simulink model "LPV_controller_Simulation_6DOF"  (R2015a)
settings: Solver=ode1  StartTime=0.0  StopTime=1.5  FixedStep=0.001  RelTol=1e-3
undefined symbols (not defined in the file): dKLFR_sim, inert, phi_mid, phi_range, rho_bnd, robot3DOFaffineLPVparams, theta_bnd, theta_mid, theta_range, Xdsim
libraries: simulink x4
settings Model: Creator=Micha  LastModifiedBy=Micha

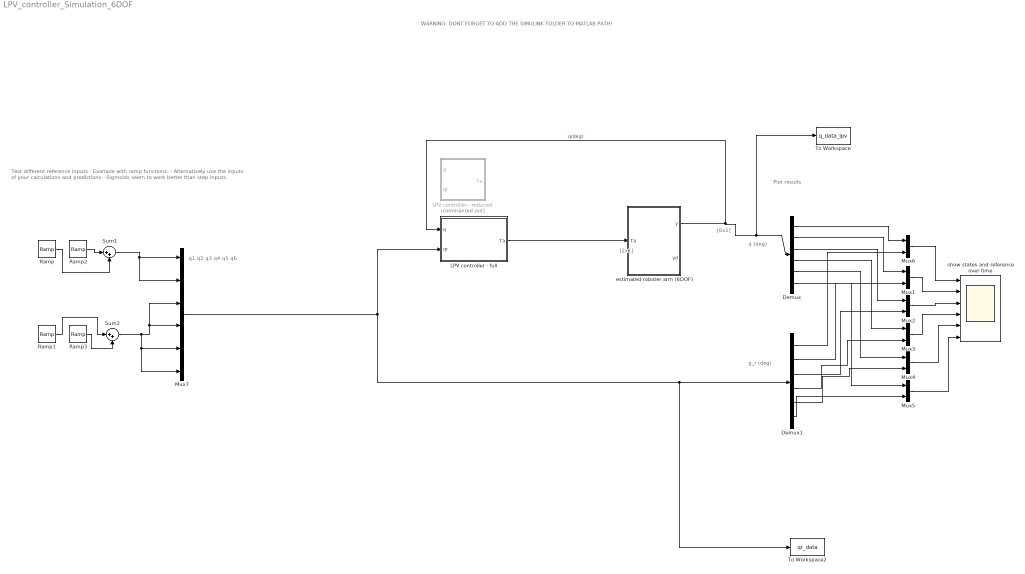
== system LPV_controller_Simulation_6DOF ==
  note: WARNING: DONT FORGET TO ADD THE SIMULINK FOLDER TO MATLAB PATH!
  note: Test different reference inputs - Example with ramp functions.
      | - Alternatively use the inputs of your calculations and predictions
      | - Sigmoids seem to work better than step inputs.
  note: [6x1]
  note: Plot results
  note: g_r (deg)
  note: [2x1]
  note: q (deg)
  note: q1
      |
      |
      | q2
      |
      |
      |
      | q3
      |
      |
      |
      |
      | q4
      |
      |
      |
      | q5
      |
      |
      |
      | q6
  Demux : Demux  Outputs=6
  Demux1 : Demux  Outputs=6
  LPV controller - full : Subsystem
  LPV controller - reduced : Subsystem  Commented=on
  Mux{1..6} (6 alike) : Mux  Inputs=2
  Mux7 : Mux  Inputs=6
  Ramp : simulink/Sources/Ramp  slope=-80  start=0.1  X0=0
  Ramp1 : simulink/Sources/Ramp  slope=60  start=0.1  X0=0
  Ramp2 : simulink/Sources/Ramp  slope=80  start=0.6  X0=0
  Ramp3 : simulink/Sources/Ramp  slope=-60  start=1  X0=0
  Sum1 : Sum  Inputs=|++
  Sum2 : Sum  Inputs=|++
  To Workspace : ToWorkspace  VariableName=q_data_lpv  SaveFormat=Timeseries  SampleTime=-1
  To Workspace2 : ToWorkspace  VariableName=qr_data  SaveFormat=Timeseries  SampleTime=-1
  "estimated roboter arm (6DOF) " : Subsystem
  show states and reference over time : Scope  NumInputPorts=6
      settings: YMin=-45~-45~10~5~5~5  YMax=-10~-10~55~55~55~55
  wires:
  Demux/1 -> Mux6/1
  Demux/2 -> Mux1/1
  Demux/3 -> Mux2/1
  Demux/4 -> Mux3/1
  Demux/5 -> Mux4/1
  Demux/6 -> Mux5/1
  Mux6/1 -> show states and reference over time/1
  Mux1/1 -> show states and reference over time/2
  Mux2/1 -> show states and reference over time/3
  Mux3/1 -> show states and reference over time/4
  Mux4/1 -> show states and reference over time/5
  Mux5/1 -> show states and reference over time/6
  Demux1/1 -> Mux6/2
  Demux1/2 -> Mux1/2
  Demux1/3 -> Mux2/2
  Demux1/4 -> Mux3/2
  Demux1/5 -> Mux4/2
  Demux1/6 -> Mux5/2
  Mux7/1 -> Demux1/1, To Workspace2/1, LPV controller - full/2(qr)
  LPV controller - full/1(Ta) -> "estimated roboter arm (6DOF) "/1(Ta)
  Ramp2/1 -> Sum1/1
  Ramp/1 -> Sum1/2
  Ramp1/1 -> Sum2/1
  Ramp3/1 -> Sum2/2
  Sum2/1 -> Mux7/6, Mux7/5, Mux7/4, Mux7/3
  Sum1/1 -> Mux7/1, Mux7/2
  "estimated roboter arm (6DOF) "/1(y) -> To Workspace/1, Demux/1, LPV controller - full/1(q)  "q(deg)"

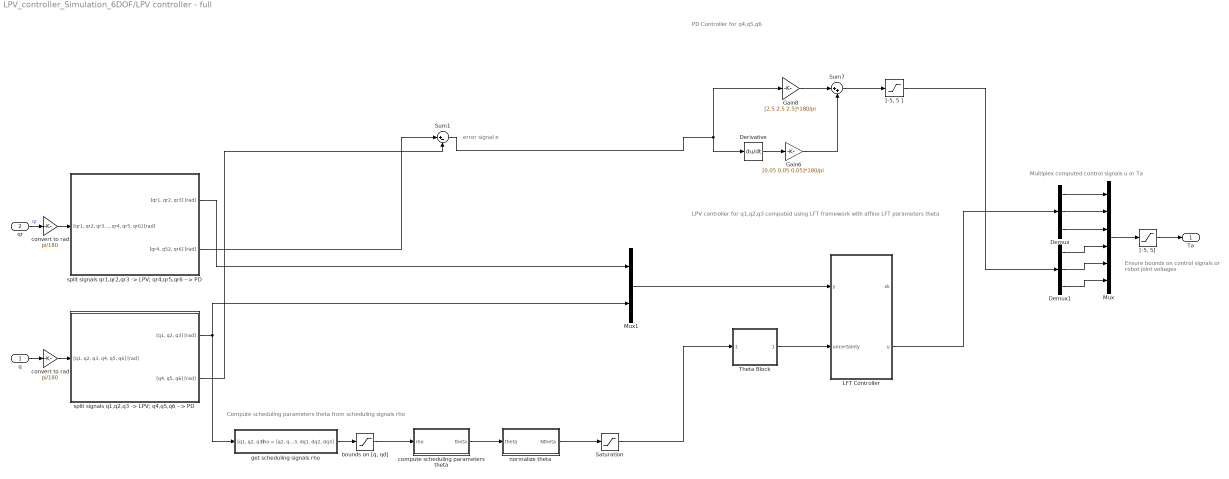
== system LPV_controller_Simulation_6DOF/LPV controller - full ==
  note: Ensure bounds on control signals
      |  or robot joint voltages
  note: Multiplex computed control signals u or Ta
  note: Compute scheduling parameters theta from scheduling signals rho
  note: error signal e
  note: LPV controller for q1,q2,q3 computed using LFT framework
      | with affine LFT parameters theta
  note: PD Controller for q4,q5,q6
  q : Inport
  qr : Inport  Port=2
  Demux : Demux  Outputs=3
  Demux1 : Demux  Outputs=3
  Derivative : Derivative
  Gain6 : Gain  Gain=[0.05 0.05 0.05]*180/pi
      settings: AttributesFormatString=D gain
  Gain8 : Gain  Gain=[2.5 2.5 2.5]*180/pi
      settings: AttributesFormatString=P gain
  LFT Controller : Subsystem  mask{P=dKLFR_sim}
      mask prompts: P "Plant"
      mask Display:
      | port_label('output', 1, 'xk')
      | port_label('output', 2, 'u')
      | port_label('input' , 1, 'e')
      | port_label('input' , 2, 'phi')
      | fprintf('Controller')
  Mux : Mux  Inputs=6
  Mux1 : Mux  Inputs=2
  Saturation : Saturate  UpperLimit=1  LowerLimit=-1
  Sum1 : Sum  Inputs=|+-
  Sum7 : Sum  Inputs=|++
  Theta Block : Subsystem
      mask Display:
      | patch([0.2 .5 0.8], [0.2 0.8 0.2], [0 0 0])
      | patch([0.25 .5 0.75], [0.25 0.75 0.25], [1 1 1])
  "[-5, 5 ]" : Saturate  UpperLimit=5  LowerLimit=-5
  "[-5, 5]" : Saturate  UpperLimit=5  LowerLimit=-5
  "bounds on [q, qd]" : Saturate  UpperLimit=rho_bnd(:, 2)  LowerLimit=rho_bnd(:, 1)
  compute scheduling parameters theta : Subsystem
  convert to rad : Gain  Gain=pi/180
  convert to rad : Gain  Gain=pi/180
  get scheduling signals rho : Subsystem
  normalize theta : Subsystem
  "split signals q1,q2,q3 -> LPV; q4,q5,q6 --> PD" : Subsystem
  "split signals qr1,qr2,qr3 -> LPV; qr4,qr5,qr6 --> PD" : Subsystem
  Ta : Outport
  wires:
  q/1 -> convert to rad/1
  qr/1 -> convert to rad/1  "qr"
  convert to rad/1 -> "split signals q1,q2,q3 -> LPV; q4,q5,q6 --> PD"/1("[q1, q2, q3, q4, q5, q6] [rad]")
  convert to rad/1 -> "split signals qr1,qr2,qr3 -> LPV; qr4,qr5,qr6 --> PD"/1("[qr1, qr2, qr3, qr4, qr5, qr6] [rad]")
  "split signals q1,q2,q3 -> LPV; q4,q5,q6 --> PD"/1("[q1, q2, q3] [rad]") -> get scheduling signals rho/1("[q1, q2, q3]"), Mux1/2
  LFT Controller/2(u) -> Demux/1
  Mux1/1 -> LFT Controller/1(y)
  Demux/1 -> Mux/1
  Demux/2 -> Mux/2
  "split signals qr1,qr2,qr3 -> LPV; qr4,qr5,qr6 --> PD"/1("[qr1, qr2, qr3] [rad]") -> Mux1/1
  get scheduling signals rho/1("rho = [q2, q3, dq1, dq2, dq3]") -> "bounds on [q, qd]"/1
  Saturation/1 -> Theta Block/1(Scheduling Parameter Vector)
  "bounds on [q, qd]"/1 -> compute scheduling parameters theta/1(rho)
  Mux/1 -> "[-5, 5]"/1
  "[-5, 5]"/1 -> Ta/1
  Demux/3 -> Mux/3
  compute scheduling parameters theta/1(theta) -> normalize theta/1(theta)
  normalize theta/1(Ntheta) -> Saturation/1
  Theta Block/1(Delta Block Vector) -> LFT Controller/2(uncertainty)
  Gain8/1 -> Sum7/1
  Derivative/1 -> Gain6/1
  Gain6/1 -> Sum7/2
  Sum1/1 -> Gain8/1, Derivative/1
  Sum7/1 -> "[-5, 5 ]"/1
  "split signals q1,q2,q3 -> LPV; q4,q5,q6 --> PD"/2("[q4, q5, q6] [rad]") -> Sum1/2
  "[-5, 5 ]"/1 -> Demux1/1
  "split signals qr1,qr2,qr3 -> LPV; qr4,qr5,qr6 --> PD"/2("[qr4, q52, qr6] [rad]") -> Sum1/1
  Demux1/1 -> Mux/4
  Demux1/2 -> Mux/5
  Demux1/3 -> Mux/6

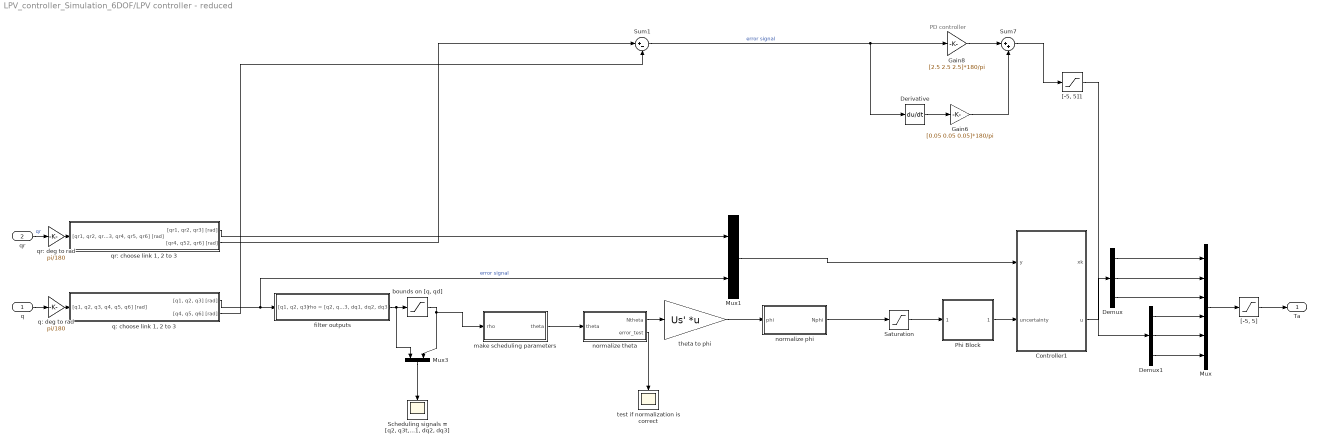
== system LPV_controller_Simulation_6DOF/LPV controller - reduced ==
  note: PD controller
  q : Inport
  qr : Inport  Port=2
  Controller1 : Subsystem  mask{P=dKLFR_sim}
      mask prompts: P "Plant"
      mask Display:
      | port_label('output', 1, 'xk')
      | port_label('output', 2, 'u')
      | port_label('input' , 1, 'e')
      | port_label('input' , 2, 'phi')
      | fprintf('Controller')
  Demux : Demux  Outputs=3
  Demux1 : Demux  Outputs=3
  Derivative : Derivative
  Gain6 : Gain  Gain=[0.05 0.05 0.05]*180/pi
      settings: AttributesFormatString=D gain
  Gain8 : Gain  Gain=[2.5 2.5 2.5]*180/pi
      settings: AttributesFormatString=P gain
  Mux : Mux  Inputs=6
  Mux1 : Mux  Inputs=2
  Mux3 : Mux  Inputs=2
  Phi Block : Subsystem
      mask Display:
      | patch([0.2 .5 0.8], [0.2 0.8 0.2], [0 0 0])
      | patch([0.25 .5 0.75], [0.25 0.75 0.25], [1 1 1])
  Saturation : Saturate  UpperLimit=1  LowerLimit=-1
  "Scheduling signals = [q2, q3t, dq1, dq2, dq3]" : Scope
      settings: ShowLegends=on  YMin=-1.75  YMax=1.5  SaveName=ScopeData2
  Sum1 : Sum  Inputs=|+-
  Sum7 : Sum  Inputs=|++
  "[-5, 5]" : Saturate  UpperLimit=5  LowerLimit=-5
  "[-5, 5]1" : Saturate  UpperLimit=5  LowerLimit=-5
  "bounds on [q, qd]" : Saturate  UpperLimit=rho_bnd(:, 2)  LowerLimit=rho_bnd(:, 1)
  filter outputs : Subsystem
  make scheduling parameters : Subsystem
  normalize phi : Subsystem
  normalize theta : Subsystem
  "q: choose link 1, 2 to 3" : Subsystem
  q: deg to rad : Gain  Gain=pi/180
  "qr: choose link 1, 2 to 3" : Subsystem
  qr: deg to rad : Gain  Gain=pi/180
  test if normalization is correct : Scope
      settings: ShowLegends=on  YMin=-1.75  YMax=1.5
  theta to phi : Gain  Gain=Us'  Multiplication=Matrix(K*u) (u vector)
  Ta : Outport
  wires:
  q/1 -> q: deg to rad/1
  qr/1 -> qr: deg to rad/1  "qr"
  q: deg to rad/1 -> "q: choose link 1, 2 to 3"/1("[q1, q2, q3, q4, q5, q6] [rad]")
  qr: deg to rad/1 -> "qr: choose link 1, 2 to 3"/1("[qr1, qr2, qr3, qr4, qr5, qr6] [rad]")
  "q: choose link 1, 2 to 3"/1("[q1, q2, q3] [rad]") -> Mux1/2, filter outputs/1("[q1, q2, q3]")  "error signal"
  Controller1/2(u) -> Demux/1
  Mux1/1 -> Controller1/1(y)
  Demux/1 -> Mux/1
  Demux/2 -> Mux/2
  "qr: choose link 1, 2 to 3"/1("[qr1, qr2, qr3] [rad]") -> Mux1/1
  filter outputs/1("rho = [q2, q3, dq1, dq2, dq3]") -> "bounds on [q, qd]"/1, Mux3/1
  Saturation/1 -> Phi Block/1(Scheduling Parameter Vector)
  "bounds on [q, qd]"/1 -> make scheduling parameters/1(rho), Mux3/2
  Mux3/1 -> "Scheduling signals = [q2, q3t, dq1, dq2, dq3]"/1
  Mux/1 -> "[-5, 5]"/1
  "[-5, 5]"/1 -> Ta/1
  Demux/3 -> Mux/3
  make scheduling parameters/1(theta) -> normalize theta/1(theta)
  normalize theta/1(Ntheta) -> theta to phi/1
  normalize theta/2(error_test) -> test if normalization is correct/1
  Phi Block/1(Delta Block Vector) -> Controller1/2(uncertainty)
  Gain8/1 -> Sum7/1
  Derivative/1 -> Gain6/1
  Gain6/1 -> Sum7/2
  Sum1/1 -> Derivative/1, Gain8/1  "error signal"
  Sum7/1 -> "[-5, 5]1"/1
  "q: choose link 1, 2 to 3"/2("[q4, q5, q6] [rad]") -> Sum1/2
  "[-5, 5]1"/1 -> Demux1/1
  "qr: choose link 1, 2 to 3"/2("[qr4, q52, qr6] [rad]") -> Sum1/1
  Demux1/1 -> Mux/4
  Demux1/2 -> Mux/5
  Demux1/3 -> Mux/6
  normalize phi/1(Nphi) -> Saturation/1
  theta to phi/1 -> normalize phi/1(phi)

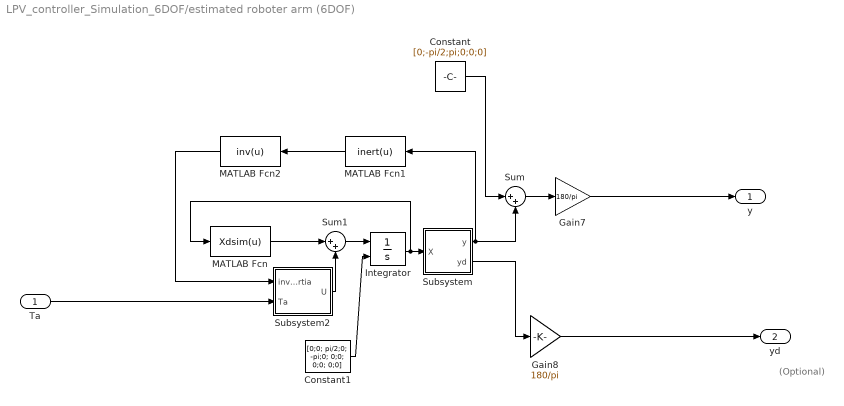
== system LPV_controller_Simulation_6DOF/estimated roboter arm (6DOF)  ==
  note: (Optional)
  Ta : Inport
  Constant : Constant  Value=[0;-pi/2;pi;0;0;0]
  Constant1 : Constant  Value="[0;0;    pi/2;0;    -pi;0;    0;0;    0;0;    0;0]"
      settings: AttributesFormatString=initial states, ready position
  Gain7 : Gain  Gain=180/pi
  Gain8 : Gain  Gain=180/pi
  Integrator : Integrator  InitialConditionSource=external
  MATLAB Fcn : MATLABFcn  MATLABFcn=Xdsim(u)
  MATLAB Fcn1 : MATLABFcn  MATLABFcn=inert(u)  Output1D=off
  MATLAB Fcn2 : MATLABFcn  MATLABFcn=inv(u)  Output1D=off
  Subsystem : Subsystem
  Subsystem2 : Subsystem
  Sum : Sum  Inputs=|++
  Sum1 : Sum  Inputs=|++
  y : Outport
  yd : Outport  Port=2
  wires:
  Sum/1 -> Gain7/1
  Constant/1 -> Sum/1
  Constant1/1 -> Integrator/2
  Integrator/1 -> MATLAB Fcn/1, Subsystem/1(X)
  Subsystem/2(yd) -> Gain8/1
  Subsystem/1(y) -> MATLAB Fcn1/1, Sum/2
  Sum1/1 -> Integrator/1
  MATLAB Fcn/1 -> Sum1/1
  Subsystem2/1("U ") -> Sum1/2
  MATLAB Fcn2/1 -> Subsystem2/1(inv inertia)
  Gain8/1 -> yd/1
  Gain7/1 -> y/1
  MATLAB Fcn1/1 -> MATLAB Fcn2/1
  Ta/1 -> Subsystem2/2(Ta)

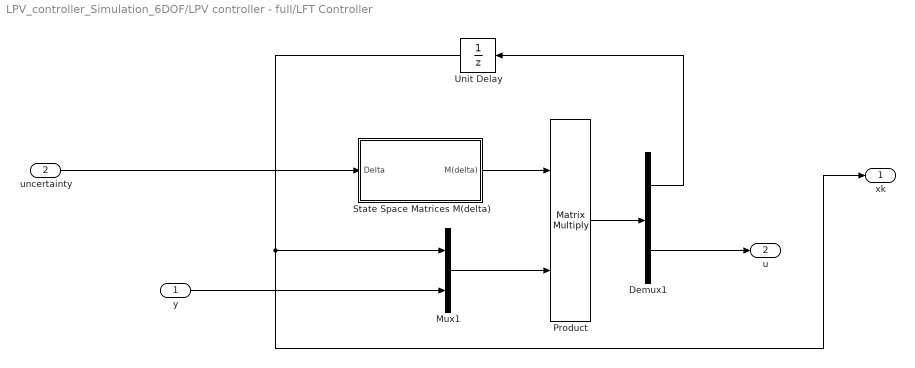
== system LPV_controller_Simulation_6DOF/LPV controller - full/LFT Controller ==
  y : Inport
  uncertainty : Inport  Port=2
  Demux1 : Demux  Outputs=[size(P.A, 1); size(P.C_y, 1)]
  Mux1 : Mux  Inputs=2
  Product : Product  Multiplication=Matrix(*)  RndMeth=Zero
  State Space Matrices M(delta) : Subsystem
  Unit Delay : UnitDelay  SampleTime=-1
  xk : Outport
  u : Outport  Port=2
  wires:
  y/1 -> Mux1/2
  Demux1/2 -> u/1
  Unit Delay/1 -> Mux1/1, xk/1
  Demux1/1 -> Unit Delay/1
  Product/1 -> Demux1/1
  Mux1/1 -> Product/2
  State Space Matrices M(delta)/1(M(delta)) -> Product/1
  uncertainty/1 -> State Space Matrices M(delta)/1(Delta)

== system LPV_controller_Simulation_6DOF/LPV controller - full/Theta Block ==
  Scheduling Parameter Vector : Inport
  MATLAB Function : MATLAB Function  TreatAsAtomicUnit=on
  Delta Block Vector : Outport
  wires:
  MATLAB Function/1(Delta) -> Delta Block Vector/1
  Scheduling Parameter Vector/1 -> MATLAB Function/1(DeltaVector)

== system LPV_controller_Simulation_6DOF/LPV controller - full/compute scheduling parameters theta ==
  rho : Inport
  MATLAB Fcn1 : MATLABFcn  MATLABFcn=robot3DOFaffineLPVparams(u)  Output1D=off
  Transpose : Math  Operator=transpose  SaturateOnIntegerOverflow=on
  theta : Outport
  wires:
  rho/1 -> Transpose/1
  MATLAB Fcn1/1 -> theta/1
  Transpose/1 -> MATLAB Fcn1/1

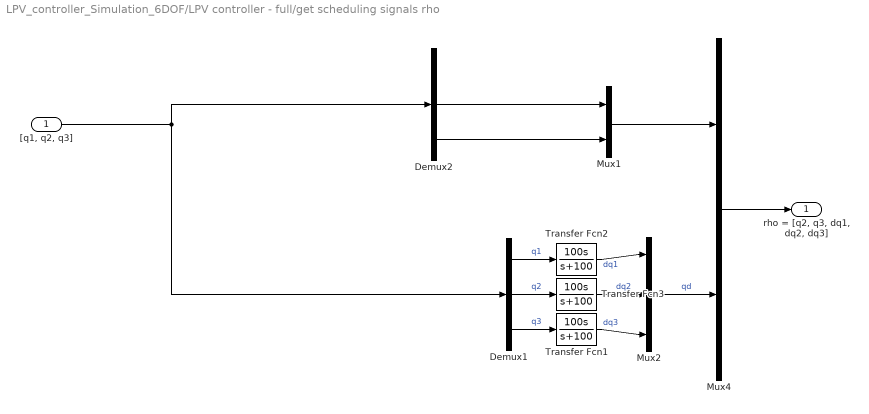
== system LPV_controller_Simulation_6DOF/LPV controller - full/get scheduling signals rho ==
  "[q1, q2, q3]" : Inport
  Demux1 : Demux  Outputs=3
  Demux2 : Demux  Outputs=3
  Mux1 : Mux  Inputs=2
  Mux2 : Mux  Inputs=3
  Mux4 : Mux  Inputs=2
  Transfer Fcn1 : TransferFcn  Numerator=[100 0]  Denominator=[1 100]
  Transfer Fcn2 : TransferFcn  Numerator=[100 0]  Denominator=[1 100]
  Transfer Fcn3 : TransferFcn  Numerator=[100 0]  Denominator=[1 100]
  "rho = [q2, q3, dq1, dq2, dq3]" : Outport
  wires:
  Mux2/1 -> Mux4/2  "qd"
  Mux4/1 -> "rho = [q2, q3, dq1, dq2, dq3]"/1
  Demux1/2 -> Transfer Fcn3/1  "q2"
  Transfer Fcn3/1 -> Mux2/2  "dq2"
  Transfer Fcn2/1 -> Mux2/1  "dq1"
  Demux1/1 -> Transfer Fcn2/1  "q1"
  "[q1, q2, q3]"/1 -> Demux1/1, Demux2/1
  Demux1/3 -> Transfer Fcn1/1  "q3"
  Transfer Fcn1/1 -> Mux2/3  "dq3"
  Demux2/2 -> Mux1/1
  Demux2/3 -> Mux1/2
  Mux1/1 -> Mux4/1

== system LPV_controller_Simulation_6DOF/LPV controller - full/normalize theta ==
  note: Normalizing is done via the following formula with y=theta and ymin = -1, ymax = 1
      |
      | y = (ymax-ymin)*(x-xmin)/(xmax-xmin) + ymin;
  theta : Inport
  Gain : Gain  Gain=2
  Gain1 : Gain  Gain=1./theta_range
  Sum : Sum  Inputs=|+-
  theta_bnd : Constant  Value=theta_mid
  Ntheta : Outport
  wires:
  Gain1/1 -> Ntheta/1
  theta/1 -> Sum/1
  theta_bnd/1 -> Sum/2
  Sum/1 -> Gain/1
  Gain/1 -> Gain1/1

== system LPV_controller_Simulation_6DOF/LPV controller - full/split signals q1,q2,q3 -> LPV; q4,q5,q6 --> PD ==
  "[q1, q2, q3, q4, q5, q6] [rad]" : Inport
  Demux : Demux  Outputs=6
  Mux : Mux  Inputs=3
  Mux1 : Mux  Inputs=3
  "[q1, q2, q3] [rad]" : Outport
  "[q4, q5, q6] [rad]" : Outport  Port=2
  wires:
  "[q1, q2, q3, q4, q5, q6] [rad]"/1 -> Demux/1
  Mux1/1 -> "[q1, q2, q3] [rad]"/1
  Demux/4 -> Mux/1
  Demux/6 -> Mux/3
  Demux/5 -> Mux/2
  Mux/1 -> "[q4, q5, q6] [rad]"/1
  Demux/3 -> Mux1/3
  Demux/2 -> Mux1/2
  Demux/1 -> Mux1/1

== system LPV_controller_Simulation_6DOF/LPV controller - full/split signals qr1,qr2,qr3 -> LPV; qr4,qr5,qr6 --> PD ==
  "[qr1, qr2, qr3, qr4, qr5, qr6] [rad]" : Inport
  Demux : Demux  Outputs=6
  Mux : Mux  Inputs=3
  Mux1 : Mux  Inputs=3
  "[qr1, qr2, qr3] [rad]" : Outport
  "[qr4, q52, qr6] [rad]" : Outport  Port=2
  wires:
  "[qr1, qr2, qr3, qr4, qr5, qr6] [rad]"/1 -> Demux/1
  Mux/1 -> "[qr1, qr2, qr3] [rad]"/1
  Demux/3 -> Mux/3
  Demux/1 -> Mux/1
  Demux/2 -> Mux/2
  Demux/4 -> Mux1/1
  Demux/5 -> Mux1/2
  Demux/6 -> Mux1/3
  Mux1/1 -> "[qr4, q52, qr6] [rad]"/1

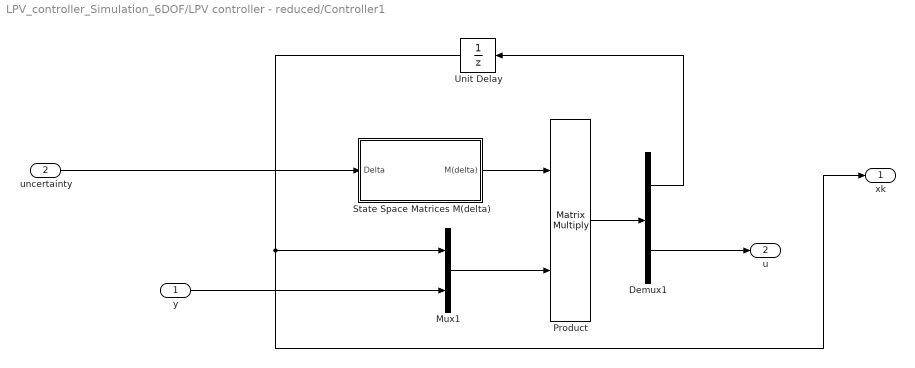
== system LPV_controller_Simulation_6DOF/LPV controller - reduced/Controller1 ==
  y : Inport
  uncertainty : Inport  Port=2
  Demux1 : Demux  Outputs=[size(P.A, 1); size(P.C_y, 1)]
  Mux1 : Mux  Inputs=2
  Product : Product  Multiplication=Matrix(*)  RndMeth=Zero
  State Space Matrices M(delta) : Subsystem
  Unit Delay : UnitDelay  SampleTime=-1
  xk : Outport
  u : Outport  Port=2
  wires:
  y/1 -> Mux1/2
  Demux1/2 -> u/1
  Unit Delay/1 -> Mux1/1, xk/1
  Demux1/1 -> Unit Delay/1
  Product/1 -> Demux1/1
  Mux1/1 -> Product/2
  State Space Matrices M(delta)/1(M(delta)) -> Product/1
  uncertainty/1 -> State Space Matrices M(delta)/1(Delta)

== system LPV_controller_Simulation_6DOF/LPV controller - reduced/Phi Block ==
  Scheduling Parameter Vector : Inport
  MATLAB Function : MATLAB Function  TreatAsAtomicUnit=on
  Delta Block Vector : Outport
  wires:
  MATLAB Function/1(PHI) -> Delta Block Vector/1
  Scheduling Parameter Vector/1 -> MATLAB Function/1(phiVector)

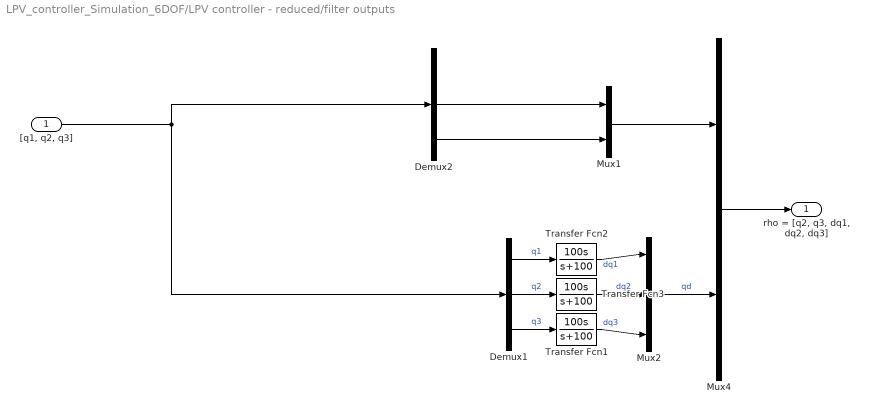
== system LPV_controller_Simulation_6DOF/LPV controller - reduced/filter outputs ==
  "[q1, q2, q3]" : Inport
  Demux1 : Demux  Outputs=3
  Demux2 : Demux  Outputs=3
  Mux1 : Mux  Inputs=2
  Mux2 : Mux  Inputs=3
  Mux4 : Mux  Inputs=2
  Transfer Fcn1 : TransferFcn  Numerator=[100 0]  Denominator=[1 100]
  Transfer Fcn2 : TransferFcn  Numerator=[100 0]  Denominator=[1 100]
  Transfer Fcn3 : TransferFcn  Numerator=[100 0]  Denominator=[1 100]
  "rho = [q2, q3, dq1, dq2, dq3]" : Outport
  wires:
  Mux2/1 -> Mux4/2  "qd"
  Mux4/1 -> "rho = [q2, q3, dq1, dq2, dq3]"/1
  Demux1/2 -> Transfer Fcn3/1  "q2"
  Transfer Fcn3/1 -> Mux2/2  "dq2"
  Transfer Fcn2/1 -> Mux2/1  "dq1"
  Demux1/1 -> Transfer Fcn2/1  "q1"
  "[q1, q2, q3]"/1 -> Demux1/1, Demux2/1
  Demux1/3 -> Transfer Fcn1/1  "q3"
  Transfer Fcn1/1 -> Mux2/3  "dq3"
  Demux2/2 -> Mux1/1
  Demux2/3 -> Mux1/2
  Mux1/1 -> Mux4/1

== system LPV_controller_Simulation_6DOF/LPV controller - reduced/make scheduling parameters ==
  rho : Inport
  MATLAB Fcn1 : MATLABFcn  MATLABFcn=robot3DOFaffineLPVparams(u)  Output1D=off
  Transpose : Math  Operator=transpose  SaturateOnIntegerOverflow=on
  theta : Outport
  wires:
  rho/1 -> Transpose/1
  MATLAB Fcn1/1 -> theta/1
  Transpose/1 -> MATLAB Fcn1/1

== system LPV_controller_Simulation_6DOF/LPV controller - reduced/normalize phi ==
  phi : Inport
  Gain : Gain  Gain=2
  Gain1 : Gain  Gain=1./phi_range
  Sum : Sum  Inputs=|+-
  theta_bnd : Constant  Value=phi_mid
  Nphi : Outport
  wires:
  Gain/1 -> Gain1/1
  Sum/1 -> Gain/1
  theta_bnd/1 -> Sum/2
  Gain1/1 -> Nphi/1
  phi/1 -> Sum/1

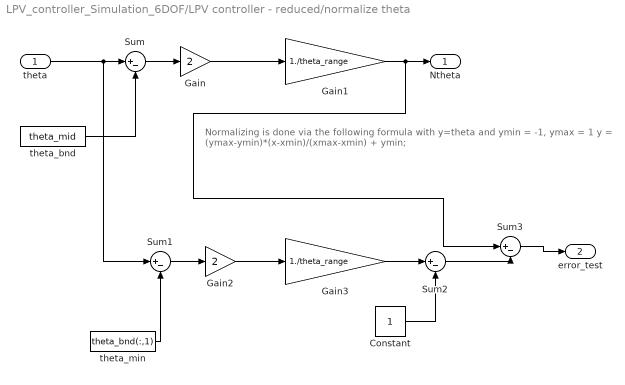
== system LPV_controller_Simulation_6DOF/LPV controller - reduced/normalize theta ==
  note: Normalizing is done via the following formula with y=theta and ymin = -1, ymax = 1
      |
      | y = (ymax-ymin)*(x-xmin)/(xmax-xmin) + ymin;
  theta : Inport
  Constant : Constant
  Gain : Gain  Gain=2
  Gain1 : Gain  Gain=1./theta_range
  Gain2 : Gain  Gain=2
  Gain3 : Gain  Gain=1./theta_range
  Sum{,1..3} (4 alike) : Sum  Inputs=|+-
  theta_bnd : Constant  Value=theta_mid
  theta_min : Constant  Value=theta_bnd(:,1)
  Ntheta : Outport
  error_test : Outport  Port=2
  wires:
  Gain1/1 -> Sum3/1, Ntheta/1
  theta/1 -> Sum1/1, Sum/1
  theta_bnd/1 -> Sum/2
  Sum/1 -> Gain/1
  Gain/1 -> Gain1/1
  theta_min/1 -> Sum1/2
  Sum1/1 -> Gain2/1
  Gain2/1 -> Gain3/1
  Gain3/1 -> Sum2/1
  Constant/1 -> Sum2/2
  Sum2/1 -> Sum3/2
  Sum3/1 -> error_test/1

== system LPV_controller_Simulation_6DOF/LPV controller - reduced/q: choose link 1, 2 to 3 ==
  "[q1, q2, q3, q4, q5, q6] [rad]" : Inport
  Demux : Demux  Outputs=6
  Mux : Mux  Inputs=3
  Mux1 : Mux  Inputs=3
  "[q1, q2, q3] [rad]" : Outport
  "[q4, q5, q6] [rad]" : Outport  Port=2
  wires:
  "[q1, q2, q3, q4, q5, q6] [rad]"/1 -> Demux/1
  Mux1/1 -> "[q1, q2, q3] [rad]"/1
  Demux/4 -> Mux/1
  Demux/6 -> Mux/3
  Demux/5 -> Mux/2
  Mux/1 -> "[q4, q5, q6] [rad]"/1
  Demux/3 -> Mux1/3
  Demux/2 -> Mux1/2
  Demux/1 -> Mux1/1

== system LPV_controller_Simulation_6DOF/LPV controller - reduced/qr: choose link 1, 2 to 3 ==
  "[qr1, qr2, qr3, qr4, qr5, qr6] [rad]" : Inport
  Demux : Demux  Outputs=6
  Mux : Mux  Inputs=3
  Mux1 : Mux  Inputs=3
  "[qr1, qr2, qr3] [rad]" : Outport
  "[qr4, q52, qr6] [rad]" : Outport  Port=2
  wires:
  "[qr1, qr2, qr3, qr4, qr5, qr6] [rad]"/1 -> Demux/1
  Mux/1 -> "[qr1, qr2, qr3] [rad]"/1
  Demux/3 -> Mux/3
  Demux/1 -> Mux/1
  Demux/2 -> Mux/2
  Demux/4 -> Mux1/1
  Demux/5 -> Mux1/2
  Demux/6 -> Mux1/3
  Mux1/1 -> "[qr4, q52, qr6] [rad]"/1

== system LPV_controller_Simulation_6DOF/estimated roboter arm (6DOF) /Subsystem ==
  X : Inport
  Demux : Demux  Outputs=12
  Mux : Mux  Inputs=6
  Mux1 : Mux  Inputs=6
  y : Outport
  yd : Outport  Port=2
  wires:
  Demux/2 -> Mux1/1
  Demux/4 -> Mux1/2
  Demux/6 -> Mux1/3
  Demux/8 -> Mux1/4
  Demux/10 -> Mux1/5
  Demux/12 -> Mux1/6
  Demux/11 -> Mux/6
  Demux/9 -> Mux/5
  Demux/7 -> Mux/4
  Demux/5 -> Mux/3
  Demux/3 -> Mux/2
  Demux/1 -> Mux/1
  Mux/1 -> y/1
  Mux1/1 -> yd/1
  X/1 -> Demux/1

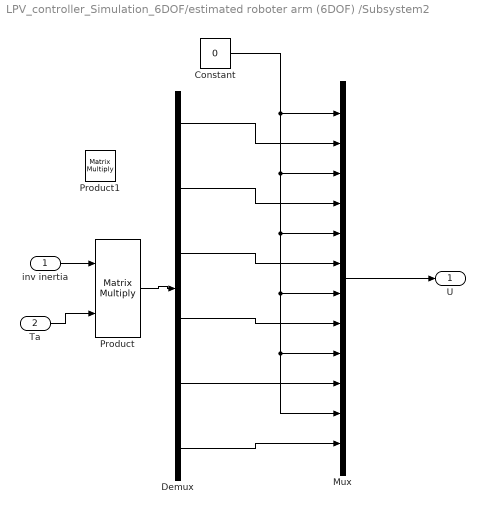
== system LPV_controller_Simulation_6DOF/estimated roboter arm (6DOF) /Subsystem2 ==
  inv inertia : Inport
  Ta : Inport  Port=2
  Constant : Constant  Value=0
  Demux : Demux  Outputs=6
  Mux : Mux  Inputs=12
  Product : Product  Multiplication=Matrix(*)  RndMeth=Zero
  Product1 : Product  Multiplication=Matrix(*)
  "U " : Outport
  wires:
  Constant/1 -> Mux/11, Mux/9, Mux/7, Mux/5, Mux/3, Mux/1
  Demux/6 -> Mux/12
  Demux/5 -> Mux/10
  Demux/4 -> Mux/8
  Demux/3 -> Mux/6
  Demux/2 -> Mux/4
  Demux/1 -> Mux/2
  Ta/1 -> Product/2
  inv inertia/1 -> Product/1
  Mux/1 -> "U "/1
  Product/1 -> Demux/1

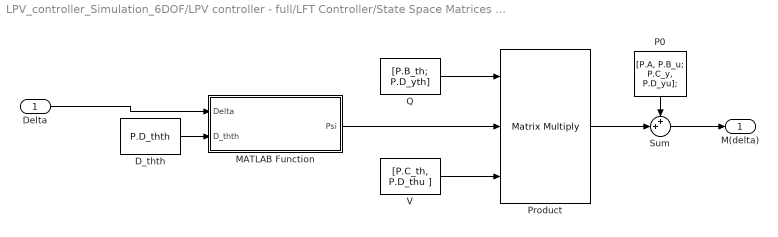
== system LPV_controller_Simulation_6DOF/LPV controller - full/LFT Controller/State Space Matrices M(delta) ==
  Delta : Inport
  D_thth : Constant  Value=P.D_thth
  MATLAB Function : MATLAB Function  TreatAsAtomicUnit=on
  P0 : Constant  Value=[P.A, P.B_u; P.C_y, P.D_yu];  VectorParams1D=off
  Product : Product  Inputs=3  Multiplication=Matrix(*)  RndMeth=Zero
  Q : Constant  Value=[P.B_th; P.D_yth]
  Sum : Sum  Inputs=++|
  V : Constant  Value=[P.C_th, P.D_thu ]  VectorParams1D=off
  M(delta) : Outport
  wires:
  MATLAB Function/1(Psi) -> Product/2
  Delta/1 -> MATLAB Function/1(Delta)
  V/1 -> Product/3
  Sum/1 -> M(delta)/1
  P0/1 -> Sum/1
  Product/1 -> Sum/2
  Q/1 -> Product/1
  D_thth/1 -> MATLAB Function/2(D_thth)

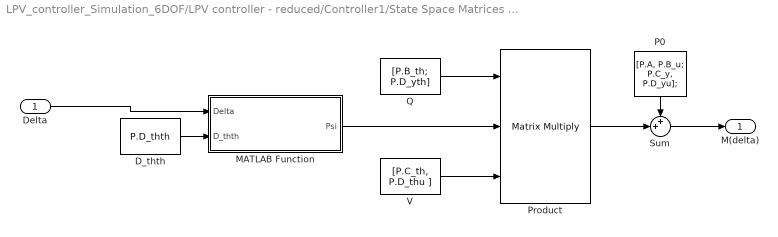
== system LPV_controller_Simulation_6DOF/LPV controller - reduced/Controller1/State Space Matrices M(delta) ==
  Delta : Inport
  D_thth : Constant  Value=P.D_thth
  MATLAB Function : MATLAB Function  TreatAsAtomicUnit=on
  P0 : Constant  Value=[P.A, P.B_u; P.C_y, P.D_yu];  VectorParams1D=off
  Product : Product  Inputs=3  Multiplication=Matrix(*)  RndMeth=Zero
  Q : Constant  Value=[P.B_th; P.D_yth]
  Sum : Sum  Inputs=++|
  V : Constant  Value=[P.C_th, P.D_thu ]  VectorParams1D=off
  M(delta) : Outport
  wires:
  MATLAB Function/1(Psi) -> Product/2
  Delta/1 -> MATLAB Function/1(Delta)
  V/1 -> Product/3
  Sum/1 -> M(delta)/1
  P0/1 -> Sum/1
  Product/1 -> Sum/2
  Q/1 -> Product/1
  D_thth/1 -> MATLAB Function/2(D_thth)

== matlab function LPV_controller_Simulation_6DOF/LPV controller - full/LFT Controller/State Space Matrices M(delta)/MATLAB Function ==
  data: Delta input; Psi output; D_thth input
function Psi = Psi(Delta, D_thth)
%#codegen

[nwth, nzth] = size(Delta);

Psi = Delta * (eye(nwth) - D_thth*Delta)^-1;

== matlab function LPV_controller_Simulation_6DOF/LPV controller - reduced/Controller1/State Space Matrices M(delta)/MATLAB Function ==
  data: Delta input; Psi output; D_thth input
function Psi = Psi(Delta, D_thth)
%#codegen

[nwth, nzth] = size(Delta);

Psi = Delta * (eye(nwth) - D_thth*Delta)^-1;

== matlab function LPV_controller_Simulation_6DOF/LPV controller - full/Theta Block/MATLAB Function ==
  data: Delta output; DeltaVector input
function Delta = Delta(DeltaVector)
%#codegen
Delta = diag(DeltaVector);

== matlab function LPV_controller_Simulation_6DOF/LPV controller - reduced/Phi Block/MATLAB Function ==
  data: PHI output; phiVector input
function PHI = PhiBlk(phiVector)
%#codegen
PHI = diag([ones(3,1)*phiVector(1); ones(3,1)*phiVector(2); ones(3,1)*phiVector(3)]);
